simulink library "LibDBC_SCU_ch1"  (R2024b)
settings: Solver=VariableStepAuto  StartTime=0.0  StopTime=10.0  RelTol=1e-3
undefined symbols (not defined in the file): bit_packing, bit_unpacking, IO_Blk_Lib_TTC500, IO_CAN_ConfigMsg, IO_CAN_ReadMsg
libraries: simulink x59, IOBlock_Library_TTC580 x32
(part 16 of 21)

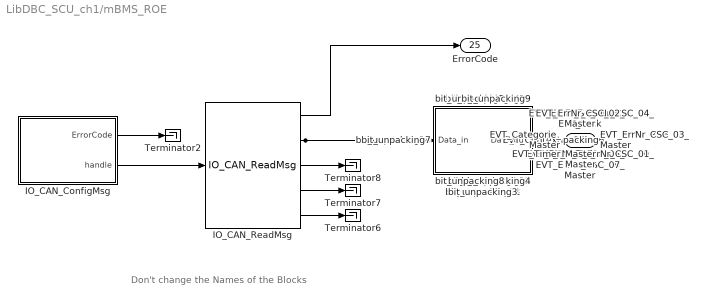
== system LibDBC_SCU_ch1/mBMS_ROE ==
  note: Don't change the Names of the Blocks
  IO_CAN_ConfigMsg : Subsystem  mask(IO_CAN_ConfigMsg_Code){SampleTime=-1, ttlib=IO_Blk_Lib_TTC500, ttDescription=IO_CAN_ConfigMsg, tt_iolib_version=0.19, channel=IO_CAN_CHANNEL_1, mode=IO_CAN_MSG_READ, id_format=IO_CAN_STD_FRAME, id=0x102, ac_mask=0x7FF}
      mask help: Configures a message object for the given CAN channel.
      mask init:
      | %
      mask Help: web(which('IO_CAN.h'))
      mask TypeOptions channel: IO_CAN_CHANNEL_0  | IO_CAN_CHANNEL_1 | IO_CAN_CHANNEL_2 | IO_CAN_CHANNEL_3 | IO_CAN_CHANNEL_4 | IO_CAN_CHANNEL_5 | IO_CAN_CHANNEL_6
      mask Callback channel: %
      mask TypeOptions mode: IO_CAN_MSG_READ | IO_CAN_MSG_WRITE
      mask Callback mode: %
      mask TypeOptions id_format: IO_CAN_STD_FRAME | IO_CAN_EXT_FRAME
      mask Callback id_format: %
      mask Callback id: %
      mask Callback ac_mask: %
  IO_CAN_ReadMsg : IOBlock_Library_TTC580/CAN  Blocks TTC580 IOlib/ReadMsg_CAN/IO_CAN_ReadMsg  SampleTime=-1  ttlib=IO_Blk_Lib_TTC500  ttDescription=IO_CAN_ReadMsg  tt_iolib_version=0.19
      settings: SourceProductName=I/O Blocklibrary for TTC580
  Terminator{2,6..8} (4 alike) : Terminator
  bit_unpacking1 : Subsystem  LoadFcn=|  mask(bit_unpacking_Code){SampleTime=-1, ttlib=IO_Blk_Lib_TTC500, ttDescription=bit_unpacking, tt_iolib_version=0.26, Endianness=little, Format=unsigned, Inversion=off, Startbit=0, Width_bits=5, Factor=1, Offset=0}
      | try
      | %
      | %Upgrade Information - standard BEGIN
      | new_color = 'blue';
      | new_ver = '0.26';
      | act_ver = get_param(gcb,'tt_iolib_version');
      | if not(strcmp(act_ver,new_ver))
      |     disp(['Upgrade block: ',gcb,char(10),'       Version: ',act_ver,' to ',new_ver]);
      |     %switch - case for specific upgrade information e.g. additional parameter required 
      |     %Change appearance and version information
      |     set_param(gcb,'ForegroundColor',new_color);
      |     set_param(gcb,'tt_iolib_version',new_ver);
      | end
      | %Upgrade Information - standard END
      | catch
      | %Standard catch section BEGIN
      | errordlg('An error occurred in a callback of the TTC580-BlockLib. Please open the Diagnostic Viewer for further details');
      | disp(' ');
      | disp('------------------------------------------------------------');
      | disp('An error occurred in a callback of the TTC580-BlockLib.');
      | disp(['Please check the parameters in the mask of ',gcb]);
      | disp('If you do not encounter any violations, then please '); 
      | disp('copy the following lines and report this to support@ttcontrol.com ');
      | disp('<< begin of error message dump >>');
      | disp(['Version of TTC580-BlockLib: ', get_param(gcb,'tt_iolib_version')]);
      | disp(get_param(gcb,'ttDescription'));
      | disp(gcb);
      | x=lasterror;disp(x.message);
      | disp(get_param(gcb,'MaskValues'));
      | disp(version);
      | disp(computer);
      | disp('<< end of error message dump >>');
      | disp('------------------------------------------------------------');
      | disp(' ');
      | %Standard catch section END
      | end
      mask help:
      | Block to read in CAN signal from a specified position within 64bit field.
      | For "Factor" and "Offset" the definition of Vector's CANdb applies:
      | [Physical value] = ( [Raw value] * [Factor] ) + [Offset]
      | with Raw value of a signal being the value as it is transmitted in the CAN-network
      | Verification capabilities are supported.
      mask init: same as LibDBC_SCU_ch1/EXT_BalancingRequest/bit_packing1
      mask Help: web([which('usermanual.html'),'#',lower(get_param(gcb,'ttDescription'))])
      mask TypeOptions Endianness: big | little
      mask Callback Endianness: %
      mask TypeOptions Format: unsigned | signed | real32
      mask Callback Format: %
      mask Callback Inversion: %
      mask Callback Startbit: %
      mask Callback Width_bits: %
      mask Callback Factor: %
      mask Callback Offset: %
  bit_unpacking10 : Subsystem  LoadFcn=|  mask(bit_unpacking_Code){SampleTime=-1, ttlib=IO_Blk_Lib_TTC500, ttDescription=bit_unpacking, tt_iolib_version=0.26, Endianness=little, Format=unsigned, Inversion=off, Startbit=8, Width_bits=8, Factor=1, Offset=0}
      | try
      | %
      | %Upgrade Information - standard BEGIN
      | new_color = 'blue';
      | new_ver = '0.26';
      | act_ver = get_param(gcb,'tt_iolib_version');
      | if not(strcmp(act_ver,new_ver))
      |     disp(['Upgrade block: ',gcb,char(10),'       Version: ',act_ver,' to ',new_ver]);
      |     %switch - case for specific upgrade information e.g. additional parameter required 
      |     %Change appearance and version information
      |     set_param(gcb,'ForegroundColor',new_color);
      |     set_param(gcb,'tt_iolib_version',new_ver);
      | end
      | %Upgrade Information - standard END
      | catch
      | %Standard catch section BEGIN
      | errordlg('An error occurred in a callback of the TTC580-BlockLib. Please open the Diagnostic Viewer for further details');
      | disp(' ');
      | disp('------------------------------------------------------------');
      | disp('An error occurred in a callback of the TTC580-BlockLib.');
      | disp(['Please check the parameters in the mask of ',gcb]);
      | disp('If you do not encounter any violations, then please '); 
      | disp('copy the following lines and report this to support@ttcontrol.com ');
      | disp('<< begin of error message dump >>');
      | disp(['Version of TTC580-BlockLib: ', get_param(gcb,'tt_iolib_version')]);
      | disp(get_param(gcb,'ttDescription'));
      | disp(gcb);
      | x=lasterror;disp(x.message);
      | disp(get_param(gcb,'MaskValues'));
      | disp(version);
      | disp(computer);
      | disp('<< end of error message dump >>');
      | disp('------------------------------------------------------------');
      | disp(' ');
      | %Standard catch section END
      | end
      mask help:
      | Block to read in CAN signal from a specified position within 64bit field.
      | For "Factor" and "Offset" the definition of Vector's CANdb applies:
      | [Physical value] = ( [Raw value] * [Factor] ) + [Offset]
      | with Raw value of a signal being the value as it is transmitted in the CAN-network
      | Verification capabilities are supported.
      mask init: same as LibDBC_SCU_ch1/EXT_BalancingRequest/bit_packing1
      mask Help: web([which('usermanual.html'),'#',lower(get_param(gcb,'ttDescription'))])
      mask TypeOptions Endianness: big | little
      mask Callback Endianness: %
      mask TypeOptions Format: unsigned | signed | real32
      mask Callback Format: %
      mask Callback Inversion: %
      mask Callback Startbit: %
      mask Callback Width_bits: %
      mask Callback Factor: %
      mask Callback Offset: %
  bit_unpacking11 : Subsystem  LoadFcn=|  mask(bit_unpacking_Code){SampleTime=-1, ttlib=IO_Blk_Lib_TTC500, ttDescription=bit_unpacking, tt_iolib_version=0.26, Endianness=little, Format=unsigned, Inversion=off, Startbit=8, Width_bits=8, Factor=1, Offset=0}
      | try
      | %
      | %Upgrade Information - standard BEGIN
      | new_color = 'blue';
      | new_ver = '0.26';
      | act_ver = get_param(gcb,'tt_iolib_version');
      | if not(strcmp(act_ver,new_ver))
      |     disp(['Upgrade block: ',gcb,char(10),'       Version: ',act_ver,' to ',new_ver]);
      |     %switch - case for specific upgrade information e.g. additional parameter required 
      |     %Change appearance and version information
      |     set_param(gcb,'ForegroundColor',new_color);
      |     set_param(gcb,'tt_iolib_version',new_ver);
      | end
      | %Upgrade Information - standard END
      | catch
      | %Standard catch section BEGIN
      | errordlg('An error occurred in a callback of the TTC580-BlockLib. Please open the Diagnostic Viewer for further details');
      | disp(' ');
      | disp('------------------------------------------------------------');
      | disp('An error occurred in a callback of the TTC580-BlockLib.');
      | disp(['Please check the parameters in the mask of ',gcb]);
      | disp('If you do not encounter any violations, then please '); 
      | disp('copy the following lines and report this to support@ttcontrol.com ');
      | disp('<< begin of error message dump >>');
      | disp(['Version of TTC580-BlockLib: ', get_param(gcb,'tt_iolib_version')]);
      | disp(get_param(gcb,'ttDescription'));
      | disp(gcb);
      | x=lasterror;disp(x.message);
      | disp(get_param(gcb,'MaskValues'));
      | disp(version);
      | disp(computer);
      | disp('<< end of error message dump >>');
      | disp('------------------------------------------------------------');
      | disp(' ');
      | %Standard catch section END
      | end
      mask help:
      | Block to read in CAN signal from a specified position within 64bit field.
      | For "Factor" and "Offset" the definition of Vector's CANdb applies:
      | [Physical value] = ( [Raw value] * [Factor] ) + [Offset]
      | with Raw value of a signal being the value as it is transmitted in the CAN-network
      | Verification capabilities are supported.
      mask init: same as LibDBC_SCU_ch1/EXT_BalancingRequest/bit_packing1
      mask Help: web([which('usermanual.html'),'#',lower(get_param(gcb,'ttDescription'))])
      mask TypeOptions Endianness: big | little
      mask Callback Endianness: %
      mask TypeOptions Format: unsigned | signed | real32
      mask Callback Format: %
      mask Callback Inversion: %
      mask Callback Startbit: %
      mask Callback Width_bits: %
      mask Callback Factor: %
      mask Callback Offset: %
  bit_unpacking12 : Subsystem  LoadFcn=|  mask(bit_unpacking_Code){SampleTime=-1, ttlib=IO_Blk_Lib_TTC500, ttDescription=bit_unpacking, tt_iolib_version=0.26, Endianness=little, Format=unsigned, Inversion=off, Startbit=8, Width_bits=8, Factor=1, Offset=0}
      | try
      | %
      | %Upgrade Information - standard BEGIN
      | new_color = 'blue';
      | new_ver = '0.26';
      | act_ver = get_param(gcb,'tt_iolib_version');
      | if not(strcmp(act_ver,new_ver))
      |     disp(['Upgrade block: ',gcb,char(10),'       Version: ',act_ver,' to ',new_ver]);
      |     %switch - case for specific upgrade information e.g. additional parameter required 
      |     %Change appearance and version information
      |     set_param(gcb,'ForegroundColor',new_color);
      |     set_param(gcb,'tt_iolib_version',new_ver);
      | end
      | %Upgrade Information - standard END
      | catch
      | %Standard catch section BEGIN
      | errordlg('An error occurred in a callback of the TTC580-BlockLib. Please open the Diagnostic Viewer for further details');
      | disp(' ');
      | disp('------------------------------------------------------------');
      | disp('An error occurred in a callback of the TTC580-BlockLib.');
      | disp(['Please check the parameters in the mask of ',gcb]);
      | disp('If you do not encounter any violations, then please '); 
      | disp('copy the following lines and report this to support@ttcontrol.com ');
      | disp('<< begin of error message dump >>');
      | disp(['Version of TTC580-BlockLib: ', get_param(gcb,'tt_iolib_version')]);
      | disp(get_param(gcb,'ttDescription'));
      | disp(gcb);
      | x=lasterror;disp(x.message);
      | disp(get_param(gcb,'MaskValues'));
      | disp(version);
      | disp(computer);
      | disp('<< end of error message dump >>');
      | disp('------------------------------------------------------------');
      | disp(' ');
      | %Standard catch section END
      | end
      mask help:
      | Block to read in CAN signal from a specified position within 64bit field.
      | For "Factor" and "Offset" the definition of Vector's CANdb applies:
      | [Physical value] = ( [Raw value] * [Factor] ) + [Offset]
      | with Raw value of a signal being the value as it is transmitted in the CAN-network
      | Verification capabilities are supported.
      mask init: same as LibDBC_SCU_ch1/EXT_BalancingRequest/bit_packing1
      mask Help: web([which('usermanual.html'),'#',lower(get_param(gcb,'ttDescription'))])
      mask TypeOptions Endianness: big | little
      mask Callback Endianness: %
      mask TypeOptions Format: unsigned | signed | real32
      mask Callback Format: %
      mask Callback Inversion: %
      mask Callback Startbit: %
      mask Callback Width_bits: %
      mask Callback Factor: %
      mask Callback Offset: %
  bit_unpacking13 : Subsystem  LoadFcn=|  mask(bit_unpacking_Code){SampleTime=-1, ttlib=IO_Blk_Lib_TTC500, ttDescription=bit_unpacking, tt_iolib_version=0.26, Endianness=little, Format=unsigned, Inversion=off, Startbit=8, Width_bits=8, Factor=1, Offset=0}
      | try
      | %
      | %Upgrade Information - standard BEGIN
      | new_color = 'blue';
      | new_ver = '0.26';
      | act_ver = get_param(gcb,'tt_iolib_version');
      | if not(strcmp(act_ver,new_ver))
      |     disp(['Upgrade block: ',gcb,char(10),'       Version: ',act_ver,' to ',new_ver]);
      |     %switch - case for specific upgrade information e.g. additional parameter required 
      |     %Change appearance and version information
      |     set_param(gcb,'ForegroundColor',new_color);
      |     set_param(gcb,'tt_iolib_version',new_ver);
      | end
      | %Upgrade Information - standard END
      | catch
      | %Standard catch section BEGIN
      | errordlg('An error occurred in a callback of the TTC580-BlockLib. Please open the Diagnostic Viewer for further details');
      | disp(' ');
      | disp('------------------------------------------------------------');
      | disp('An error occurred in a callback of the TTC580-BlockLib.');
      | disp(['Please check the parameters in the mask of ',gcb]);
      | disp('If you do not encounter any violations, then please '); 
      | disp('copy the following lines and report this to support@ttcontrol.com ');
      | disp('<< begin of error message dump >>');
      | disp(['Version of TTC580-BlockLib: ', get_param(gcb,'tt_iolib_version')]);
      | disp(get_param(gcb,'ttDescription'));
      | disp(gcb);
      | x=lasterror;disp(x.message);
      | disp(get_param(gcb,'MaskValues'));
      | disp(version);
      | disp(computer);
      | disp('<< end of error message dump >>');
      | disp('------------------------------------------------------------');
      | disp(' ');
      | %Standard catch section END
      | end
      mask help:
      | Block to read in CAN signal from a specified position within 64bit field.
      | For "Factor" and "Offset" the definition of Vector's CANdb applies:
      | [Physical value] = ( [Raw value] * [Factor] ) + [Offset]
      | with Raw value of a signal being the value as it is transmitted in the CAN-network
      | Verification capabilities are supported.
      mask init: same as LibDBC_SCU_ch1/EXT_BalancingRequest/bit_packing1
      mask Help: web([which('usermanual.html'),'#',lower(get_param(gcb,'ttDescription'))])
      mask TypeOptions Endianness: big | little
      mask Callback Endianness: %
      mask TypeOptions Format: unsigned | signed | real32
      mask Callback Format: %
      mask Callback Inversion: %
      mask Callback Startbit: %
      mask Callback Width_bits: %
      mask Callback Factor: %
      mask Callback Offset: %
  bit_unpacking14 : Subsystem  LoadFcn=|  mask(bit_unpacking_Code){SampleTime=-1, ttlib=IO_Blk_Lib_TTC500, ttDescription=bit_unpacking, tt_iolib_version=0.26, Endianness=little, Format=unsigned, Inversion=off, Startbit=8, Width_bits=8, Factor=1, Offset=0}
      | try
      | %
      | %Upgrade Information - standard BEGIN
      | new_color = 'blue';
      | new_ver = '0.26';
      | act_ver = get_param(gcb,'tt_iolib_version');
      | if not(strcmp(act_ver,new_ver))
      |     disp(['Upgrade block: ',gcb,char(10),'       Version: ',act_ver,' to ',new_ver]);
      |     %switch - case for specific upgrade information e.g. additional parameter required 
      |     %Change appearance and version information
      |     set_param(gcb,'ForegroundColor',new_color);
      |     set_param(gcb,'tt_iolib_version',new_ver);
      | end
      | %Upgrade Information - standard END
      | catch
      | %Standard catch section BEGIN
      | errordlg('An error occurred in a callback of the TTC580-BlockLib. Please open the Diagnostic Viewer for further details');
      | disp(' ');
      | disp('------------------------------------------------------------');
      | disp('An error occurred in a callback of the TTC580-BlockLib.');
      | disp(['Please check the parameters in the mask of ',gcb]);
      | disp('If you do not encounter any violations, then please '); 
      | disp('copy the following lines and report this to support@ttcontrol.com ');
      | disp('<< begin of error message dump >>');
      | disp(['Version of TTC580-BlockLib: ', get_param(gcb,'tt_iolib_version')]);
      | disp(get_param(gcb,'ttDescription'));
      | disp(gcb);
      | x=lasterror;disp(x.message);
      | disp(get_param(gcb,'MaskValues'));
      | disp(version);
      | disp(computer);
      | disp('<< end of error message dump >>');
      | disp('------------------------------------------------------------');
      | disp(' ');
      | %Standard catch section END
      | end
      mask help:
      | Block to read in CAN signal from a specified position within 64bit field.
      | For "Factor" and "Offset" the definition of Vector's CANdb applies:
      | [Physical value] = ( [Raw value] * [Factor] ) + [Offset]
      | with Raw value of a signal being the value as it is transmitted in the CAN-network
      | Verification capabilities are supported.
      mask init: same as LibDBC_SCU_ch1/EXT_BalancingRequest/bit_packing1
      mask Help: web([which('usermanual.html'),'#',lower(get_param(gcb,'ttDescription'))])
      mask TypeOptions Endianness: big | little
      mask Callback Endianness: %
      mask TypeOptions Format: unsigned | signed | real32
      mask Callback Format: %
      mask Callback Inversion: %
      mask Callback Startbit: %
      mask Callback Width_bits: %
      mask Callback Factor: %
      mask Callback Offset: %
  bit_unpacking15 : Subsystem  LoadFcn=|  mask(bit_unpacking_Code){SampleTime=-1, ttlib=IO_Blk_Lib_TTC500, ttDescription=bit_unpacking, tt_iolib_version=0.26, Endianness=little, Format=unsigned, Inversion=off, Startbit=8, Width_bits=8, Factor=1, Offset=0}
      | try
      | %
      | %Upgrade Information - standard BEGIN
      | new_color = 'blue';
      | new_ver = '0.26';
      | act_ver = get_param(gcb,'tt_iolib_version');
      | if not(strcmp(act_ver,new_ver))
      |     disp(['Upgrade block: ',gcb,char(10),'       Version: ',act_ver,' to ',new_ver]);
      |     %switch - case for specific upgrade information e.g. additional parameter required 
      |     %Change appearance and version information
      |     set_param(gcb,'ForegroundColor',new_color);
      |     set_param(gcb,'tt_iolib_version',new_ver);
      | end
      | %Upgrade Information - standard END
      | catch
      | %Standard catch section BEGIN
      | errordlg('An error occurred in a callback of the TTC580-BlockLib. Please open the Diagnostic Viewer for further details');
      | disp(' ');
      | disp('------------------------------------------------------------');
      | disp('An error occurred in a callback of the TTC580-BlockLib.');
      | disp(['Please check the parameters in the mask of ',gcb]);
      | disp('If you do not encounter any violations, then please '); 
      | disp('copy the following lines and report this to support@ttcontrol.com ');
      | disp('<< begin of error message dump >>');
      | disp(['Version of TTC580-BlockLib: ', get_param(gcb,'tt_iolib_version')]);
      | disp(get_param(gcb,'ttDescription'));
      | disp(gcb);
      | x=lasterror;disp(x.message);
      | disp(get_param(gcb,'MaskValues'));
      | disp(version);
      | disp(computer);
      | disp('<< end of error message dump >>');
      | disp('------------------------------------------------------------');
      | disp(' ');
      | %Standard catch section END
      | end
      mask help:
      | Block to read in CAN signal from a specified position within 64bit field.
      | For "Factor" and "Offset" the definition of Vector's CANdb applies:
      | [Physical value] = ( [Raw value] * [Factor] ) + [Offset]
      | with Raw value of a signal being the value as it is transmitted in the CAN-network
      | Verification capabilities are supported.
      mask init: same as LibDBC_SCU_ch1/EXT_BalancingRequest/bit_packing1
      mask Help: web([which('usermanual.html'),'#',lower(get_param(gcb,'ttDescription'))])
      mask TypeOptions Endianness: big | little
      mask Callback Endianness: %
      mask TypeOptions Format: unsigned | signed | real32
      mask Callback Format: %
      mask Callback Inversion: %
      mask Callback Startbit: %
      mask Callback Width_bits: %
      mask Callback Factor: %
      mask Callback Offset: %
  bit_unpacking16 : Subsystem  LoadFcn=|  mask(bit_unpacking_Code){SampleTime=-1, ttlib=IO_Blk_Lib_TTC500, ttDescription=bit_unpacking, tt_iolib_version=0.26, Endianness=little, Format=unsigned, Inversion=off, Startbit=8, Width_bits=8, Factor=1, Offset=0}
      | try
      | %
      | %Upgrade Information - standard BEGIN
      | new_color = 'blue';
      | new_ver = '0.26';
      | act_ver = get_param(gcb,'tt_iolib_version');
      | if not(strcmp(act_ver,new_ver))
      |     disp(['Upgrade block: ',gcb,char(10),'       Version: ',act_ver,' to ',new_ver]);
      |     %switch - case for specific upgrade information e.g. additional parameter required 
      |     %Change appearance and version information
      |     set_param(gcb,'ForegroundColor',new_color);
      |     set_param(gcb,'tt_iolib_version',new_ver);
      | end
      | %Upgrade Information - standard END
      | catch
      | %Standard catch section BEGIN
      | errordlg('An error occurred in a callback of the TTC580-BlockLib. Please open the Diagnostic Viewer for further details');
      | disp(' ');
      | disp('------------------------------------------------------------');
      | disp('An error occurred in a callback of the TTC580-BlockLib.');
      | disp(['Please check the parameters in the mask of ',gcb]);
      | disp('If you do not encounter any violations, then please '); 
      | disp('copy the following lines and report this to support@ttcontrol.com ');
      | disp('<< begin of error message dump >>');
      | disp(['Version of TTC580-BlockLib: ', get_param(gcb,'tt_iolib_version')]);
      | disp(get_param(gcb,'ttDescription'));
      | disp(gcb);
      | x=lasterror;disp(x.message);
      | disp(get_param(gcb,'MaskValues'));
      | disp(version);
      | disp(computer);
      | disp('<< end of error message dump >>');
      | disp('------------------------------------------------------------');
      | disp(' ');
      | %Standard catch section END
      | end
      mask help:
      | Block to read in CAN signal from a specified position within 64bit field.
      | For "Factor" and "Offset" the definition of Vector's CANdb applies:
      | [Physical value] = ( [Raw value] * [Factor] ) + [Offset]
      | with Raw value of a signal being the value as it is transmitted in the CAN-network
      | Verification capabilities are supported.
      mask init: same as LibDBC_SCU_ch1/EXT_BalancingRequest/bit_packing1
      mask Help: web([which('usermanual.html'),'#',lower(get_param(gcb,'ttDescription'))])
      mask TypeOptions Endianness: big | little
      mask Callback Endianness: %
      mask TypeOptions Format: unsigned | signed | real32
      mask Callback Format: %
      mask Callback Inversion: %
      mask Callback Startbit: %
      mask Callback Width_bits: %
      mask Callback Factor: %
      mask Callback Offset: %
  bit_unpacking17 : Subsystem  LoadFcn=|  mask(bit_unpacking_Code){SampleTime=-1, ttlib=IO_Blk_Lib_TTC500, ttDescription=bit_unpacking, tt_iolib_version=0.26, Endianness=little, Format=unsigned, Inversion=off, Startbit=8, Width_bits=8, Factor=1, Offset=0}
      | try
      | %
      | %Upgrade Information - standard BEGIN
      | new_color = 'blue';
      | new_ver = '0.26';
      | act_ver = get_param(gcb,'tt_iolib_version');
      | if not(strcmp(act_ver,new_ver))
      |     disp(['Upgrade block: ',gcb,char(10),'       Version: ',act_ver,' to ',new_ver]);
      |     %switch - case for specific upgrade information e.g. additional parameter required 
      |     %Change appearance and version information
      |     set_param(gcb,'ForegroundColor',new_color);
      |     set_param(gcb,'tt_iolib_version',new_ver);
      | end
      | %Upgrade Information - standard END
      | catch
      | %Standard catch section BEGIN
      | errordlg('An error occurred in a callback of the TTC580-BlockLib. Please open the Diagnostic Viewer for further details');
      | disp(' ');
      | disp('------------------------------------------------------------');
      | disp('An error occurred in a callback of the TTC580-BlockLib.');
      | disp(['Please check the parameters in the mask of ',gcb]);
      | disp('If you do not encounter any violations, then please '); 
      | disp('copy the following lines and report this to support@ttcontrol.com ');
      | disp('<< begin of error message dump >>');
      | disp(['Version of TTC580-BlockLib: ', get_param(gcb,'tt_iolib_version')]);
      | disp(get_param(gcb,'ttDescription'));
      | disp(gcb);
      | x=lasterror;disp(x.message);
      | disp(get_param(gcb,'MaskValues'));
      | disp(version);
      | disp(computer);
      | disp('<< end of error message dump >>');
      | disp('------------------------------------------------------------');
      | disp(' ');
      | %Standard catch section END
      | end
      mask help:
      | Block to read in CAN signal from a specified position within 64bit field.
      | For "Factor" and "Offset" the definition of Vector's CANdb applies:
      | [Physical value] = ( [Raw value] * [Factor] ) + [Offset]
      | with Raw value of a signal being the value as it is transmitted in the CAN-network
      | Verification capabilities are supported.
      mask init: same as LibDBC_SCU_ch1/EXT_BalancingRequest/bit_packing1
      mask Help: web([which('usermanual.html'),'#',lower(get_param(gcb,'ttDescription'))])
      mask TypeOptions Endianness: big | little
      mask Callback Endianness: %
      mask TypeOptions Format: unsigned | signed | real32
      mask Callback Format: %
      mask Callback Inversion: %
      mask Callback Startbit: %
      mask Callback Width_bits: %
      mask Callback Factor: %
      mask Callback Offset: %
  bit_unpacking18 : Subsystem  LoadFcn=|  mask(bit_unpacking_Code){SampleTime=-1, ttlib=IO_Blk_Lib_TTC500, ttDescription=bit_unpacking, tt_iolib_version=0.26, Endianness=little, Format=unsigned, Inversion=off, Startbit=8, Width_bits=8, Factor=1, Offset=0}
      | try
      | %
      | %Upgrade Information - standard BEGIN
      | new_color = 'blue';
      | new_ver = '0.26';
      | act_ver = get_param(gcb,'tt_iolib_version');
      | if not(strcmp(act_ver,new_ver))
      |     disp(['Upgrade block: ',gcb,char(10),'       Version: ',act_ver,' to ',new_ver]);
      |     %switch - case for specific upgrade information e.g. additional parameter required 
      |     %Change appearance and version information
      |     set_param(gcb,'ForegroundColor',new_color);
      |     set_param(gcb,'tt_iolib_version',new_ver);
      | end
      | %Upgrade Information - standard END
      | catch
      | %Standard catch section BEGIN
      | errordlg('An error occurred in a callback of the TTC580-BlockLib. Please open the Diagnostic Viewer for further details');
      | disp(' ');
      | disp('------------------------------------------------------------');
      | disp('An error occurred in a callback of the TTC580-BlockLib.');
      | disp(['Please check the parameters in the mask of ',gcb]);
      | disp('If you do not encounter any violations, then please '); 
      | disp('copy the following lines and report this to support@ttcontrol.com ');
      | disp('<< begin of error message dump >>');
      | disp(['Version of TTC580-BlockLib: ', get_param(gcb,'tt_iolib_version')]);
      | disp(get_param(gcb,'ttDescription'));
      | disp(gcb);
      | x=lasterror;disp(x.message);
      | disp(get_param(gcb,'MaskValues'));
      | disp(version);
      | disp(computer);
      | disp('<< end of error message dump >>');
      | disp('------------------------------------------------------------');
      | disp(' ');
      | %Standard catch section END
      | end
      mask help:
      | Block to read in CAN signal from a specified position within 64bit field.
      | For "Factor" and "Offset" the definition of Vector's CANdb applies:
      | [Physical value] = ( [Raw value] * [Factor] ) + [Offset]
      | with Raw value of a signal being the value as it is transmitted in the CAN-network
      | Verification capabilities are supported.
      mask init: same as LibDBC_SCU_ch1/EXT_BalancingRequest/bit_packing1
      mask Help: web([which('usermanual.html'),'#',lower(get_param(gcb,'ttDescription'))])
      mask TypeOptions Endianness: big | little
      mask Callback Endianness: %
      mask TypeOptions Format: unsigned | signed | real32
      mask Callback Format: %
      mask Callback Inversion: %
      mask Callback Startbit: %
      mask Callback Width_bits: %
      mask Callback Factor: %
      mask Callback Offset: %
  bit_unpacking19 : Subsystem  LoadFcn=|  mask(bit_unpacking_Code){SampleTime=-1, ttlib=IO_Blk_Lib_TTC500, ttDescription=bit_unpacking, tt_iolib_version=0.26, Endianness=little, Format=unsigned, Inversion=off, Startbit=8, Width_bits=8, Factor=1, Offset=0}
      | try
      | %
      | %Upgrade Information - standard BEGIN
      | new_color = 'blue';
      | new_ver = '0.26';
      | act_ver = get_param(gcb,'tt_iolib_version');
      | if not(strcmp(act_ver,new_ver))
      |     disp(['Upgrade block: ',gcb,char(10),'       Version: ',act_ver,' to ',new_ver]);
      |     %switch - case for specific upgrade information e.g. additional parameter required 
      |     %Change appearance and version information
      |     set_param(gcb,'ForegroundColor',new_color);
      |     set_param(gcb,'tt_iolib_version',new_ver);
      | end
      | %Upgrade Information - standard END
      | catch
      | %Standard catch section BEGIN
      | errordlg('An error occurred in a callback of the TTC580-BlockLib. Please open the Diagnostic Viewer for further details');
      | disp(' ');
      | disp('------------------------------------------------------------');
      | disp('An error occurred in a callback of the TTC580-BlockLib.');
      | disp(['Please check the parameters in the mask of ',gcb]);
      | disp('If you do not encounter any violations, then please '); 
      | disp('copy the following lines and report this to support@ttcontrol.com ');
      | disp('<< begin of error message dump >>');
      | disp(['Version of TTC580-BlockLib: ', get_param(gcb,'tt_iolib_version')]);
      | disp(get_param(gcb,'ttDescription'));
      | disp(gcb);
      | x=lasterror;disp(x.message);
      | disp(get_param(gcb,'MaskValues'));
      | disp(version);
      | disp(computer);
      | disp('<< end of error message dump >>');
      | disp('------------------------------------------------------------');
      | disp(' ');
      | %Standard catch section END
      | end
      mask help:
      | Block to read in CAN signal from a specified position within 64bit field.
      | For "Factor" and "Offset" the definition of Vector's CANdb applies:
      | [Physical value] = ( [Raw value] * [Factor] ) + [Offset]
      | with Raw value of a signal being the value as it is transmitted in the CAN-network
      | Verification capabilities are supported.
      mask init: same as LibDBC_SCU_ch1/EXT_BalancingRequest/bit_packing1
      mask Help: web([which('usermanual.html'),'#',lower(get_param(gcb,'ttDescription'))])
      mask TypeOptions Endianness: big | little
      mask Callback Endianness: %
      mask TypeOptions Format: unsigned | signed | real32
      mask Callback Format: %
      mask Callback Inversion: %
      mask Callback Startbit: %
      mask Callback Width_bits: %
      mask Callback Factor: %
      mask Callback Offset: %
  bit_unpacking2 : Subsystem  LoadFcn=|  mask(bit_unpacking_Code){SampleTime=-1, ttlib=IO_Blk_Lib_TTC500, ttDescription=bit_unpacking, tt_iolib_version=0.26, Endianness=little, Format=unsigned, Inversion=off, Startbit=5, Width_bits=3, Factor=1, Offset=0}
      | try
      | %
      | %Upgrade Information - standard BEGIN
      | new_color = 'blue';
      | new_ver = '0.26';
      | act_ver = get_param(gcb,'tt_iolib_version');
      | if not(strcmp(act_ver,new_ver))
      |     disp(['Upgrade block: ',gcb,char(10),'       Version: ',act_ver,' to ',new_ver]);
      |     %switch - case for specific upgrade information e.g. additional parameter required 
      |     %Change appearance and version information
      |     set_param(gcb,'ForegroundColor',new_color);
      |     set_param(gcb,'tt_iolib_version',new_ver);
      | end
      | %Upgrade Information - standard END
      | catch
      | %Standard catch section BEGIN
      | errordlg('An error occurred in a callback of the TTC580-BlockLib. Please open the Diagnostic Viewer for further details');
      | disp(' ');
      | disp('------------------------------------------------------------');
      | disp('An error occurred in a callback of the TTC580-BlockLib.');
      | disp(['Please check the parameters in the mask of ',gcb]);
      | disp('If you do not encounter any violations, then please '); 
      | disp('copy the following lines and report this to support@ttcontrol.com ');
      | disp('<< begin of error message dump >>');
      | disp(['Version of TTC580-BlockLib: ', get_param(gcb,'tt_iolib_version')]);
      | disp(get_param(gcb,'ttDescription'));
      | disp(gcb);
      | x=lasterror;disp(x.message);
      | disp(get_param(gcb,'MaskValues'));
      | disp(version);
      | disp(computer);
      | disp('<< end of error message dump >>');
      | disp('------------------------------------------------------------');
      | disp(' ');
      | %Standard catch section END
      | end
      mask help:
      | Block to read in CAN signal from a specified position within 64bit field.
      | For "Factor" and "Offset" the definition of Vector's CANdb applies:
      | [Physical value] = ( [Raw value] * [Factor] ) + [Offset]
      | with Raw value of a signal being the value as it is transmitted in the CAN-network
      | Verification capabilities are supported.
      mask init: same as LibDBC_SCU_ch1/EXT_BalancingRequest/bit_packing1
      mask Help: web([which('usermanual.html'),'#',lower(get_param(gcb,'ttDescription'))])
      mask TypeOptions Endianness: big | little
      mask Callback Endianness: %
      mask TypeOptions Format: unsigned | signed | real32
      mask Callback Format: %
      mask Callback Inversion: %
      mask Callback Startbit: %
      mask Callback Width_bits: %
      mask Callback Factor: %
      mask Callback Offset: %
  bit_unpacking20 : Subsystem  LoadFcn=|  mask(bit_unpacking_Code){SampleTime=-1, ttlib=IO_Blk_Lib_TTC500, ttDescription=bit_unpacking, tt_iolib_version=0.26, Endianness=little, Format=unsigned, Inversion=off, Startbit=8, Width_bits=8, Factor=1, Offset=0}
      | try
      | %
      | %Upgrade Information - standard BEGIN
      | new_color = 'blue';
      | new_ver = '0.26';
      | act_ver = get_param(gcb,'tt_iolib_version');
      | if not(strcmp(act_ver,new_ver))
      |     disp(['Upgrade block: ',gcb,char(10),'       Version: ',act_ver,' to ',new_ver]);
      |     %switch - case for specific upgrade information e.g. additional parameter required 
      |     %Change appearance and version information
      |     set_param(gcb,'ForegroundColor',new_color);
      |     set_param(gcb,'tt_iolib_version',new_ver);
      | end
      | %Upgrade Information - standard END
      | catch
      | %Standard catch section BEGIN
      | errordlg('An error occurred in a callback of the TTC580-BlockLib. Please open the Diagnostic Viewer for further details');
      | disp(' ');
      | disp('------------------------------------------------------------');
      | disp('An error occurred in a callback of the TTC580-BlockLib.');
      | disp(['Please check the parameters in the mask of ',gcb]);
      | disp('If you do not encounter any violations, then please '); 
      | disp('copy the following lines and report this to support@ttcontrol.com ');
      | disp('<< begin of error message dump >>');
      | disp(['Version of TTC580-BlockLib: ', get_param(gcb,'tt_iolib_version')]);
      | disp(get_param(gcb,'ttDescription'));
      | disp(gcb);
      | x=lasterror;disp(x.message);
      | disp(get_param(gcb,'MaskValues'));
      | disp(version);
      | disp(computer);
      | disp('<< end of error message dump >>');
      | disp('------------------------------------------------------------');
      | disp(' ');
      | %Standard catch section END
      | end
      mask help:
      | Block to read in CAN signal from a specified position within 64bit field.
      | For "Factor" and "Offset" the definition of Vector's CANdb applies:
      | [Physical value] = ( [Raw value] * [Factor] ) + [Offset]
      | with Raw value of a signal being the value as it is transmitted in the CAN-network
      | Verification capabilities are supported.
      mask init: same as LibDBC_SCU_ch1/EXT_BalancingRequest/bit_packing1
      mask Help: web([which('usermanual.html'),'#',lower(get_param(gcb,'ttDescription'))])
      mask TypeOptions Endianness: big | little
      mask Callback Endianness: %
      mask TypeOptions Format: unsigned | signed | real32
      mask Callback Format: %
      mask Callback Inversion: %
      mask Callback Startbit: %
      mask Callback Width_bits: %
      mask Callback Factor: %
      mask Callback Offset: %
  bit_unpacking21 : Subsystem  LoadFcn=|  mask(bit_unpacking_Code){SampleTime=-1, ttlib=IO_Blk_Lib_TTC500, ttDescription=bit_unpacking, tt_iolib_version=0.26, Endianness=little, Format=unsigned, Inversion=off, Startbit=8, Width_bits=8, Factor=1, Offset=0}
      | try
      | %
      | %Upgrade Information - standard BEGIN
      | new_color = 'blue';
      | new_ver = '0.26';
      | act_ver = get_param(gcb,'tt_iolib_version');
      | if not(strcmp(act_ver,new_ver))
      |     disp(['Upgrade block: ',gcb,char(10),'       Version: ',act_ver,' to ',new_ver]);
      |     %switch - case for specific upgrade information e.g. additional parameter required 
      |     %Change appearance and version information
      |     set_param(gcb,'ForegroundColor',new_color);
      |     set_param(gcb,'tt_iolib_version',new_ver);
      | end
      | %Upgrade Information - standard END
      | catch
      | %Standard catch section BEGIN
      | errordlg('An error occurred in a callback of the TTC580-BlockLib. Please open the Diagnostic Viewer for further details');
      | disp(' ');
      | disp('------------------------------------------------------------');
      | disp('An error occurred in a callback of the TTC580-BlockLib.');
      | disp(['Please check the parameters in the mask of ',gcb]);
      | disp('If you do not encounter any violations, then please '); 
      | disp('copy the following lines and report this to support@ttcontrol.com ');
      | disp('<< begin of error message dump >>');
      | disp(['Version of TTC580-BlockLib: ', get_param(gcb,'tt_iolib_version')]);
      | disp(get_param(gcb,'ttDescription'));
      | disp(gcb);
      | x=lasterror;disp(x.message);
      | disp(get_param(gcb,'MaskValues'));
      | disp(version);
      | disp(computer);
      | disp('<< end of error message dump >>');
      | disp('------------------------------------------------------------');
      | disp(' ');
      | %Standard catch section END
      | end
      mask help:
      | Block to read in CAN signal from a specified position within 64bit field.
      | For "Factor" and "Offset" the definition of Vector's CANdb applies:
      | [Physical value] = ( [Raw value] * [Factor] ) + [Offset]
      | with Raw value of a signal being the value as it is transmitted in the CAN-network
      | Verification capabilities are supported.
      mask init: same as LibDBC_SCU_ch1/EXT_BalancingRequest/bit_packing1
      mask Help: web([which('usermanual.html'),'#',lower(get_param(gcb,'ttDescription'))])
      mask TypeOptions Endianness: big | little
      mask Callback Endianness: %
      mask TypeOptions Format: unsigned | signed | real32
      mask Callback Format: %
      mask Callback Inversion: %
      mask Callback Startbit: %
      mask Callback Width_bits: %
      mask Callback Factor: %
      mask Callback Offset: %
  bit_unpacking22 : Subsystem  LoadFcn=|  mask(bit_unpacking_Code){SampleTime=-1, ttlib=IO_Blk_Lib_TTC500, ttDescription=bit_unpacking, tt_iolib_version=0.26, Endianness=little, Format=signed, Inversion=off, Startbit=16, Width_bits=16, Factor=1, Offset=0}
      | try
      | %
      | %Upgrade Information - standard BEGIN
      | new_color = 'blue';
      | new_ver = '0.26';
      | act_ver = get_param(gcb,'tt_iolib_version');
      | if not(strcmp(act_ver,new_ver))
      |     disp(['Upgrade block: ',gcb,char(10),'       Version: ',act_ver,' to ',new_ver]);
      |     %switch - case for specific upgrade information e.g. additional parameter required 
      |     %Change appearance and version information
      |     set_param(gcb,'ForegroundColor',new_color);
      |     set_param(gcb,'tt_iolib_version',new_ver);
      | end
      | %Upgrade Information - standard END
      | catch
      | %Standard catch section BEGIN
      | errordlg('An error occurred in a callback of the TTC580-BlockLib. Please open the Diagnostic Viewer for further details');
      | disp(' ');
      | disp('------------------------------------------------------------');
      | disp('An error occurred in a callback of the TTC580-BlockLib.');
      | disp(['Please check the parameters in the mask of ',gcb]);
      | disp('If you do not encounter any violations, then please '); 
      | disp('copy the following lines and report this to support@ttcontrol.com ');
      | disp('<< begin of error message dump >>');
      | disp(['Version of TTC580-BlockLib: ', get_param(gcb,'tt_iolib_version')]);
      | disp(get_param(gcb,'ttDescription'));
      | disp(gcb);
      | x=lasterror;disp(x.message);
      | disp(get_param(gcb,'MaskValues'));
      | disp(version);
      | disp(computer);
      | disp('<< end of error message dump >>');
      | disp('------------------------------------------------------------');
      | disp(' ');
      | %Standard catch section END
      | end
      mask help:
      | Block to read in CAN signal from a specified position within 64bit field.
      | For "Factor" and "Offset" the definition of Vector's CANdb applies:
      | [Physical value] = ( [Raw value] * [Factor] ) + [Offset]
      | with Raw value of a signal being the value as it is transmitted in the CAN-network
      | Verification capabilities are supported.
      mask init: same as LibDBC_SCU_ch1/EXT_BalancingRequest/bit_packing1
      mask Help: web([which('usermanual.html'),'#',lower(get_param(gcb,'ttDescription'))])
      mask TypeOptions Endianness: big | little
      mask Callback Endianness: %
      mask TypeOptions Format: unsigned | signed | real32
      mask Callback Format: %
      mask Callback Inversion: %
      mask Callback Startbit: %
      mask Callback Width_bits: %
      mask Callback Factor: %
      mask Callback Offset: %
  bit_unpacking23 : Subsystem  LoadFcn=|  mask(bit_unpacking_Code){SampleTime=-1, ttlib=IO_Blk_Lib_TTC500, ttDescription=bit_unpacking, tt_iolib_version=0.26, Endianness=little, Format=unsigned, Inversion=off, Startbit=32, Width_bits=2, Factor=1, Offset=0}
      | try
      | %
      | %Upgrade Information - standard BEGIN
      | new_color = 'blue';
      | new_ver = '0.26';
      | act_ver = get_param(gcb,'tt_iolib_version');
      | if not(strcmp(act_ver,new_ver))
      |     disp(['Upgrade block: ',gcb,char(10),'       Version: ',act_ver,' to ',new_ver]);
      |     %switch - case for specific upgrade information e.g. additional parameter required 
      |     %Change appearance and version information
      |     set_param(gcb,'ForegroundColor',new_color);
      |     set_param(gcb,'tt_iolib_version',new_ver);
      | end
      | %Upgrade Information - standard END
      | catch
      | %Standard catch section BEGIN
      | errordlg('An error occurred in a callback of the TTC580-BlockLib. Please open the Diagnostic Viewer for further details');
      | disp(' ');
      | disp('------------------------------------------------------------');
      | disp('An error occurred in a callback of the TTC580-BlockLib.');
      | disp(['Please check the parameters in the mask of ',gcb]);
      | disp('If you do not encounter any violations, then please '); 
      | disp('copy the following lines and report this to support@ttcontrol.com ');
      | disp('<< begin of error message dump >>');
      | disp(['Version of TTC580-BlockLib: ', get_param(gcb,'tt_iolib_version')]);
      | disp(get_param(gcb,'ttDescription'));
      | disp(gcb);
      | x=lasterror;disp(x.message);
      | disp(get_param(gcb,'MaskValues'));
      | disp(version);
      | disp(computer);
      | disp('<< end of error message dump >>');
      | disp('------------------------------------------------------------');
      | disp(' ');
      | %Standard catch section END
      | end
      mask help:
      | Block to read in CAN signal from a specified position within 64bit field.
      | For "Factor" and "Offset" the definition of Vector's CANdb applies:
      | [Physical value] = ( [Raw value] * [Factor] ) + [Offset]
      | with Raw value of a signal being the value as it is transmitted in the CAN-network
      | Verification capabilities are supported.
      mask init: same as LibDBC_SCU_ch1/EXT_BalancingRequest/bit_packing1
      mask Help: web([which('usermanual.html'),'#',lower(get_param(gcb,'ttDescription'))])
      mask TypeOptions Endianness: big | little
      mask Callback Endianness: %
      mask TypeOptions Format: unsigned | signed | real32
      mask Callback Format: %
      mask Callback Inversion: %
      mask Callback Startbit: %
      mask Callback Width_bits: %
      mask Callback Factor: %
      mask Callback Offset: %
  bit_unpacking24 : Subsystem  LoadFcn=|  mask(bit_unpacking_Code){SampleTime=-1, ttlib=IO_Blk_Lib_TTC500, ttDescription=bit_unpacking, tt_iolib_version=0.26, Endianness=little, Format=unsigned, Inversion=off, Startbit=34, Width_bits=30, Factor=1, Offset=0}
      | try
      | %
      | %Upgrade Information - standard BEGIN
      | new_color = 'blue';
      | new_ver = '0.26';
      | act_ver = get_param(gcb,'tt_iolib_version');
      | if not(strcmp(act_ver,new_ver))
      |     disp(['Upgrade block: ',gcb,char(10),'       Version: ',act_ver,' to ',new_ver]);
      |     %switch - case for specific upgrade information e.g. additional parameter required 
      |     %Change appearance and version information
      |     set_param(gcb,'ForegroundColor',new_color);
      |     set_param(gcb,'tt_iolib_version',new_ver);
      | end
      | %Upgrade Information - standard END
      | catch
      | %Standard catch section BEGIN
      | errordlg('An error occurred in a callback of the TTC580-BlockLib. Please open the Diagnostic Viewer for further details');
      | disp(' ');
      | disp('------------------------------------------------------------');
      | disp('An error occurred in a callback of the TTC580-BlockLib.');
      | disp(['Please check the parameters in the mask of ',gcb]);
      | disp('If you do not encounter any violations, then please '); 
      | disp('copy the following lines and report this to support@ttcontrol.com ');
      | disp('<< begin of error message dump >>');
      | disp(['Version of TTC580-BlockLib: ', get_param(gcb,'tt_iolib_version')]);
      | disp(get_param(gcb,'ttDescription'));
      | disp(gcb);
      | x=lasterror;disp(x.message);
      | disp(get_param(gcb,'MaskValues'));
      | disp(version);
      | disp(computer);
      | disp('<< end of error message dump >>');
      | disp('------------------------------------------------------------');
      | disp(' ');
      | %Standard catch section END
      | end
      mask help:
      | Block to read in CAN signal from a specified position within 64bit field.
      | For "Factor" and "Offset" the definition of Vector's CANdb applies:
      | [Physical value] = ( [Raw value] * [Factor] ) + [Offset]
      | with Raw value of a signal being the value as it is transmitted in the CAN-network
      | Verification capabilities are supported.
      mask init: same as LibDBC_SCU_ch1/EXT_BalancingRequest/bit_packing1
      mask Help: web([which('usermanual.html'),'#',lower(get_param(gcb,'ttDescription'))])
      mask TypeOptions Endianness: big | little
      mask Callback Endianness: %
      mask TypeOptions Format: unsigned | signed | real32
      mask Callback Format: %
      mask Callback Inversion: %
      mask Callback Startbit: %
      mask Callback Width_bits: %
      mask Callback Factor: %
      mask Callback Offset: %
  bit_unpacking3 : Subsystem  LoadFcn=|  mask(bit_unpacking_Code){SampleTime=-1, ttlib=IO_Blk_Lib_TTC500, ttDescription=bit_unpacking, tt_iolib_version=0.26, Endianness=little, Format=unsigned, Inversion=off, Startbit=8, Width_bits=8, Factor=1, Offset=0}
      | try
      | %
      | %Upgrade Information - standard BEGIN
      | new_color = 'blue';
      | new_ver = '0.26';
      | act_ver = get_param(gcb,'tt_iolib_version');
      | if not(strcmp(act_ver,new_ver))
      |     disp(['Upgrade block: ',gcb,char(10),'       Version: ',act_ver,' to ',new_ver]);
      |     %switch - case for specific upgrade information e.g. additional parameter required 
      |     %Change appearance and version information
      |     set_param(gcb,'ForegroundColor',new_color);
      |     set_param(gcb,'tt_iolib_version',new_ver);
      | end
      | %Upgrade Information - standard END
      | catch
      | %Standard catch section BEGIN
      | errordlg('An error occurred in a callback of the TTC580-BlockLib. Please open the Diagnostic Viewer for further details');
      | disp(' ');
      | disp('------------------------------------------------------------');
      | disp('An error occurred in a callback of the TTC580-BlockLib.');
      | disp(['Please check the parameters in the mask of ',gcb]);
      | disp('If you do not encounter any violations, then please '); 
      | disp('copy the following lines and report this to support@ttcontrol.com ');
      | disp('<< begin of error message dump >>');
      | disp(['Version of TTC580-BlockLib: ', get_param(gcb,'tt_iolib_version')]);
      | disp(get_param(gcb,'ttDescription'));
      | disp(gcb);
      | x=lasterror;disp(x.message);
      | disp(get_param(gcb,'MaskValues'));
      | disp(version);
      | disp(computer);
      | disp('<< end of error message dump >>');
      | disp('------------------------------------------------------------');
      | disp(' ');
      | %Standard catch section END
      | end
      mask help:
      | Block to read in CAN signal from a specified position within 64bit field.
      | For "Factor" and "Offset" the definition of Vector's CANdb applies:
      | [Physical value] = ( [Raw value] * [Factor] ) + [Offset]
      | with Raw value of a signal being the value as it is transmitted in the CAN-network
      | Verification capabilities are supported.
      mask init: same as LibDBC_SCU_ch1/EXT_BalancingRequest/bit_packing1
      mask Help: web([which('usermanual.html'),'#',lower(get_param(gcb,'ttDescription'))])
      mask TypeOptions Endianness: big | little
      mask Callback Endianness: %
      mask TypeOptions Format: unsigned | signed | real32
      mask Callback Format: %
      mask Callback Inversion: %
      mask Callback Startbit: %
      mask Callback Width_bits: %
      mask Callback Factor: %
      mask Callback Offset: %
  bit_unpacking4 : Subsystem  LoadFcn=|  mask(bit_unpacking_Code){SampleTime=-1, ttlib=IO_Blk_Lib_TTC500, ttDescription=bit_unpacking, tt_iolib_version=0.26, Endianness=little, Format=unsigned, Inversion=off, Startbit=8, Width_bits=8, Factor=1, Offset=0}
      | try
      | %
      | %Upgrade Information - standard BEGIN
      | new_color = 'blue';
      | new_ver = '0.26';
      | act_ver = get_param(gcb,'tt_iolib_version');
      | if not(strcmp(act_ver,new_ver))
      |     disp(['Upgrade block: ',gcb,char(10),'       Version: ',act_ver,' to ',new_ver]);
      |     %switch - case for specific upgrade information e.g. additional parameter required 
      |     %Change appearance and version information
      |     set_param(gcb,'ForegroundColor',new_color);
      |     set_param(gcb,'tt_iolib_version',new_ver);
      | end
      | %Upgrade Information - standard END
      | catch
      | %Standard catch section BEGIN
      | errordlg('An error occurred in a callback of the TTC580-BlockLib. Please open the Diagnostic Viewer for further details');
      | disp(' ');
      | disp('------------------------------------------------------------');
      | disp('An error occurred in a callback of the TTC580-BlockLib.');
      | disp(['Please check the parameters in the mask of ',gcb]);
      | disp('If you do not encounter any violations, then please '); 
      | disp('copy the following lines and report this to support@ttcontrol.com ');
      | disp('<< begin of error message dump >>');
      | disp(['Version of TTC580-BlockLib: ', get_param(gcb,'tt_iolib_version')]);
      | disp(get_param(gcb,'ttDescription'));
      | disp(gcb);
      | x=lasterror;disp(x.message);
      | disp(get_param(gcb,'MaskValues'));
      | disp(version);
      | disp(computer);
      | disp('<< end of error message dump >>');
      | disp('------------------------------------------------------------');
      | disp(' ');
      | %Standard catch section END
      | end
      mask help:
      | Block to read in CAN signal from a specified position within 64bit field.
      | For "Factor" and "Offset" the definition of Vector's CANdb applies:
      | [Physical value] = ( [Raw value] * [Factor] ) + [Offset]
      | with Raw value of a signal being the value as it is transmitted in the CAN-network
      | Verification capabilities are supported.
      mask init: same as LibDBC_SCU_ch1/EXT_BalancingRequest/bit_packing1
      mask Help: web([which('usermanual.html'),'#',lower(get_param(gcb,'ttDescription'))])
      mask TypeOptions Endianness: big | little
      mask Callback Endianness: %
      mask TypeOptions Format: unsigned | signed | real32
      mask Callback Format: %
      mask Callback Inversion: %
      mask Callback Startbit: %
      mask Callback Width_bits: %
      mask Callback Factor: %
      mask Callback Offset: %
  bit_unpacking5 : Subsystem  LoadFcn=|  mask(bit_unpacking_Code){SampleTime=-1, ttlib=IO_Blk_Lib_TTC500, ttDescription=bit_unpacking, tt_iolib_version=0.26, Endianness=little, Format=unsigned, Inversion=off, Startbit=8, Width_bits=8, Factor=1, Offset=0}
      | try
      | %
      | %Upgrade Information - standard BEGIN
      | new_color = 'blue';
      | new_ver = '0.26';
      | act_ver = get_param(gcb,'tt_iolib_version');
      | if not(strcmp(act_ver,new_ver))
      |     disp(['Upgrade block: ',gcb,char(10),'       Version: ',act_ver,' to ',new_ver]);
      |     %switch - case for specific upgrade information e.g. additional parameter required 
      |     %Change appearance and version information
      |     set_param(gcb,'ForegroundColor',new_color);
      |     set_param(gcb,'tt_iolib_version',new_ver);
      | end
      | %Upgrade Information - standard END
      | catch
      | %Standard catch section BEGIN
      | errordlg('An error occurred in a callback of the TTC580-BlockLib. Please open the Diagnostic Viewer for further details');
      | disp(' ');
      | disp('------------------------------------------------------------');
      | disp('An error occurred in a callback of the TTC580-BlockLib.');
      | disp(['Please check the parameters in the mask of ',gcb]);
      | disp('If you do not encounter any violations, then please '); 
      | disp('copy the following lines and report this to support@ttcontrol.com ');
      | disp('<< begin of error message dump >>');
      | disp(['Version of TTC580-BlockLib: ', get_param(gcb,'tt_iolib_version')]);
      | disp(get_param(gcb,'ttDescription'));
      | disp(gcb);
      | x=lasterror;disp(x.message);
      | disp(get_param(gcb,'MaskValues'));
      | disp(version);
      | disp(computer);
      | disp('<< end of error message dump >>');
      | disp('------------------------------------------------------------');
      | disp(' ');
      | %Standard catch section END
      | end
      mask help:
      | Block to read in CAN signal from a specified position within 64bit field.
      | For "Factor" and "Offset" the definition of Vector's CANdb applies:
      | [Physical value] = ( [Raw value] * [Factor] ) + [Offset]
      | with Raw value of a signal being the value as it is transmitted in the CAN-network
      | Verification capabilities are supported.
      mask init: same as LibDBC_SCU_ch1/EXT_BalancingRequest/bit_packing1
      mask Help: web([which('usermanual.html'),'#',lower(get_param(gcb,'ttDescription'))])
      mask TypeOptions Endianness: big | little
      mask Callback Endianness: %
      mask TypeOptions Format: unsigned | signed | real32
      mask Callback Format: %
      mask Callback Inversion: %
      mask Callback Startbit: %
      mask Callback Width_bits: %
      mask Callback Factor: %
      mask Callback Offset: %
  bit_unpacking6 : Subsystem  LoadFcn=|  mask(bit_unpacking_Code){SampleTime=-1, ttlib=IO_Blk_Lib_TTC500, ttDescription=bit_unpacking, tt_iolib_version=0.26, Endianness=little, Format=unsigned, Inversion=off, Startbit=8, Width_bits=8, Factor=1, Offset=0}
      | try
      | %
      | %Upgrade Information - standard BEGIN
      | new_color = 'blue';
      | new_ver = '0.26';
      | act_ver = get_param(gcb,'tt_iolib_version');
      | if not(strcmp(act_ver,new_ver))
      |     disp(['Upgrade block: ',gcb,char(10),'       Version: ',act_ver,' to ',new_ver]);
      |     %switch - case for specific upgrade information e.g. additional parameter required 
      |     %Change appearance and version information
      |     set_param(gcb,'ForegroundColor',new_color);
      |     set_param(gcb,'tt_iolib_version',new_ver);
      | end
      | %Upgrade Information - standard END
      | catch
      | %Standard catch section BEGIN
      | errordlg('An error occurred in a callback of the TTC580-BlockLib. Please open the Diagnostic Viewer for further details');
      | disp(' ');
      | disp('------------------------------------------------------------');
      | disp('An error occurred in a callback of the TTC580-BlockLib.');
      | disp(['Please check the parameters in the mask of ',gcb]);
      | disp('If you do not encounter any violations, then please '); 
      | disp('copy the following lines and report this to support@ttcontrol.com ');
      | disp('<< begin of error message dump >>');
      | disp(['Version of TTC580-BlockLib: ', get_param(gcb,'tt_iolib_version')]);
      | disp(get_param(gcb,'ttDescription'));
      | disp(gcb);
      | x=lasterror;disp(x.message);
      | disp(get_param(gcb,'MaskValues'));
      | disp(version);
      | disp(computer);
      | disp('<< end of error message dump >>');
      | disp('------------------------------------------------------------');
      | disp(' ');
      | %Standard catch section END
      | end
      mask help:
      | Block to read in CAN signal from a specified position within 64bit field.
      | For "Factor" and "Offset" the definition of Vector's CANdb applies:
      | [Physical value] = ( [Raw value] * [Factor] ) + [Offset]
      | with Raw value of a signal being the value as it is transmitted in the CAN-network
      | Verification capabilities are supported.
      mask init: same as LibDBC_SCU_ch1/EXT_BalancingRequest/bit_packing1
      mask Help: web([which('usermanual.html'),'#',lower(get_param(gcb,'ttDescription'))])
      mask TypeOptions Endianness: big | little
      mask Callback Endianness: %
      mask TypeOptions Format: unsigned | signed | real32
      mask Callback Format: %
      mask Callback Inversion: %
      mask Callback Startbit: %
      mask Callback Width_bits: %
      mask Callback Factor: %
      mask Callback Offset: %
  bit_unpacking7 : Subsystem  LoadFcn=|  mask(bit_unpacking_Code){SampleTime=-1, ttlib=IO_Blk_Lib_TTC500, ttDescription=bit_unpacking, tt_iolib_version=0.26, Endianness=little, Format=unsigned, Inversion=off, Startbit=8, Width_bits=8, Factor=1, Offset=0}
      | try
      | %
      | %Upgrade Information - standard BEGIN
      | new_color = 'blue';
      | new_ver = '0.26';
      | act_ver = get_param(gcb,'tt_iolib_version');
      | if not(strcmp(act_ver,new_ver))
      |     disp(['Upgrade block: ',gcb,char(10),'       Version: ',act_ver,' to ',new_ver]);
      |     %switch - case for specific upgrade information e.g. additional parameter required 
      |     %Change appearance and version information
      |     set_param(gcb,'ForegroundColor',new_color);
      |     set_param(gcb,'tt_iolib_version',new_ver);
      | end
      | %Upgrade Information - standard END
      | catch
      | %Standard catch section BEGIN
      | errordlg('An error occurred in a callback of the TTC580-BlockLib. Please open the Diagnostic Viewer for further details');
      | disp(' ');
      | disp('------------------------------------------------------------');
      | disp('An error occurred in a callback of the TTC580-BlockLib.');
      | disp(['Please check the parameters in the mask of ',gcb]);
      | disp('If you do not encounter any violations, then please '); 
      | disp('copy the following lines and report this to support@ttcontrol.com ');
      | disp('<< begin of error message dump >>');
      | disp(['Version of TTC580-BlockLib: ', get_param(gcb,'tt_iolib_version')]);
      | disp(get_param(gcb,'ttDescription'));
      | disp(gcb);
      | x=lasterror;disp(x.message);
      | disp(get_param(gcb,'MaskValues'));
      | disp(version);
      | disp(computer);
      | disp('<< end of error message dump >>');
      | disp('------------------------------------------------------------');
      | disp(' ');
      | %Standard catch section END
      | end
      mask help:
      | Block to read in CAN signal from a specified position within 64bit field.
      | For "Factor" and "Offset" the definition of Vector's CANdb applies:
      | [Physical value] = ( [Raw value] * [Factor] ) + [Offset]
      | with Raw value of a signal being the value as it is transmitted in the CAN-network
      | Verification capabilities are supported.
      mask init: same as LibDBC_SCU_ch1/EXT_BalancingRequest/bit_packing1
      mask Help: web([which('usermanual.html'),'#',lower(get_param(gcb,'ttDescription'))])
      mask TypeOptions Endianness: big | little
      mask Callback Endianness: %
      mask TypeOptions Format: unsigned | signed | real32
      mask Callback Format: %
      mask Callback Inversion: %
      mask Callback Startbit: %
      mask Callback Width_bits: %
      mask Callback Factor: %
      mask Callback Offset: %
  bit_unpacking8 : Subsystem  LoadFcn=|  mask(bit_unpacking_Code){SampleTime=-1, ttlib=IO_Blk_Lib_TTC500, ttDescription=bit_unpacking, tt_iolib_version=0.26, Endianness=little, Format=unsigned, Inversion=off, Startbit=8, Width_bits=8, Factor=1, Offset=0}
      | try
      | %
      | %Upgrade Information - standard BEGIN
      | new_color = 'blue';
      | new_ver = '0.26';
      | act_ver = get_param(gcb,'tt_iolib_version');
      | if not(strcmp(act_ver,new_ver))
      |     disp(['Upgrade block: ',gcb,char(10),'       Version: ',act_ver,' to ',new_ver]);
      |     %switch - case for specific upgrade information e.g. additional parameter required 
      |     %Change appearance and version information
      |     set_param(gcb,'ForegroundColor',new_color);
      |     set_param(gcb,'tt_iolib_version',new_ver);
      | end
      | %Upgrade Information - standard END
      | catch
      | %Standard catch section BEGIN
      | errordlg('An error occurred in a callback of the TTC580-BlockLib. Please open the Diagnostic Viewer for further details');
      | disp(' ');
      | disp('------------------------------------------------------------');
      | disp('An error occurred in a callback of the TTC580-BlockLib.');
      | disp(['Please check the parameters in the mask of ',gcb]);
      | disp('If you do not encounter any violations, then please '); 
      | disp('copy the following lines and report this to support@ttcontrol.com ');
      | disp('<< begin of error message dump >>');
      | disp(['Version of TTC580-BlockLib: ', get_param(gcb,'tt_iolib_version')]);
      | disp(get_param(gcb,'ttDescription'));
      | disp(gcb);
      | x=lasterror;disp(x.message);
      | disp(get_param(gcb,'MaskValues'));
      | disp(version);
      | disp(computer);
      | disp('<< end of error message dump >>');
      | disp('------------------------------------------------------------');
      | disp(' ');
      | %Standard catch section END
      | end
      mask help:
      | Block to read in CAN signal from a specified position within 64bit field.
      | For "Factor" and "Offset" the definition of Vector's CANdb applies:
      | [Physical value] = ( [Raw value] * [Factor] ) + [Offset]
      | with Raw value of a signal being the value as it is transmitted in the CAN-network
      | Verification capabilities are supported.
      mask init: same as LibDBC_SCU_ch1/EXT_BalancingRequest/bit_packing1
      mask Help: web([which('usermanual.html'),'#',lower(get_param(gcb,'ttDescription'))])
      mask TypeOptions Endianness: big | little
      mask Callback Endianness: %
      mask TypeOptions Format: unsigned | signed | real32
      mask Callback Format: %
      mask Callback Inversion: %
      mask Callback Startbit: %
      mask Callback Width_bits: %
      mask Callback Factor: %
      mask Callback Offset: %
  bit_unpacking9 : Subsystem  LoadFcn=|  mask(bit_unpacking_Code){SampleTime=-1, ttlib=IO_Blk_Lib_TTC500, ttDescription=bit_unpacking, tt_iolib_version=0.26, Endianness=little, Format=unsigned, Inversion=off, Startbit=8, Width_bits=8, Factor=1, Offset=0}
      | try
      | %
      | %Upgrade Information - standard BEGIN
      | new_color = 'blue';
      | new_ver = '0.26';
      | act_ver = get_param(gcb,'tt_iolib_version');
      | if not(strcmp(act_ver,new_ver))
      |     disp(['Upgrade block: ',gcb,char(10),'       Version: ',act_ver,' to ',new_ver]);
      |     %switch - case for specific upgrade information e.g. additional parameter required 
      |     %Change appearance and version information
      |     set_param(gcb,'ForegroundColor',new_color);
      |     set_param(gcb,'tt_iolib_version',new_ver);
      | end
      | %Upgrade Information - standard END
      | catch
      | %Standard catch section BEGIN
      | errordlg('An error occurred in a callback of the TTC580-BlockLib. Please open the Diagnostic Viewer for further details');
      | disp(' ');
      | disp('------------------------------------------------------------');
      | disp('An error occurred in a callback of the TTC580-BlockLib.');
      | disp(['Please check the parameters in the mask of ',gcb]);
      | disp('If you do not encounter any violations, then please '); 
      | disp('copy the following lines and report this to support@ttcontrol.com ');
      | disp('<< begin of error message dump >>');
      | disp(['Version of TTC580-BlockLib: ', get_param(gcb,'tt_iolib_version')]);
      | disp(get_param(gcb,'ttDescription'));
      | disp(gcb);
      | x=lasterror;disp(x.message);
      | disp(get_param(gcb,'MaskValues'));
      | disp(version);
      | disp(computer);
      | disp('<< end of error message dump >>');
      | disp('------------------------------------------------------------');
      | disp(' ');
      | %Standard catch section END
      | end
      mask help:
      | Block to read in CAN signal from a specified position within 64bit field.
      | For "Factor" and "Offset" the definition of Vector's CANdb applies:
      | [Physical value] = ( [Raw value] * [Factor] ) + [Offset]
      | with Raw value of a signal being the value as it is transmitted in the CAN-network
      | Verification capabilities are supported.
      mask init: same as LibDBC_SCU_ch1/EXT_BalancingRequest/bit_packing1
      mask Help: web([which('usermanual.html'),'#',lower(get_param(gcb,'ttDescription'))])
      mask TypeOptions Endianness: big | little
      mask Callback Endianness: %
      mask TypeOptions Format: unsigned | signed | real32
      mask Callback Format: %
      mask Callback Inversion: %
      mask Callback Startbit: %
      mask Callback Width_bits: %
      mask Callback Factor: %
      mask Callback Offset: %
  EVT_Component : Outport  VectorParamsAs1DForOutWhenUnconnected=off
  EVT_Pack : Outport  Port=2  VectorParamsAs1DForOutWhenUnconnected=off
  EVT_ErrNr_CSC_16_Master : Outport  Port=3  VectorParamsAs1DForOutWhenUnconnected=off
  EVT_ErrNr_CSC_15_Master : Outport  Port=4  VectorParamsAs1DForOutWhenUnconnected=off
  EVT_ErrNr_CSC_14_Master : Outport  Port=5  VectorParamsAs1DForOutWhenUnconnected=off
  EVT_ErrNr_CSC_13_Master : Outport  Port=6  VectorParamsAs1DForOutWhenUnconnected=off
  EVT_ErrNr_CSC_12_Master : Outport  Port=7  VectorParamsAs1DForOutWhenUnconnected=off
  EVT_ErrNr_CSC_11_Master : Outport  Port=8  VectorParamsAs1DForOutWhenUnconnected=off
  EVT_ErrNr_CSC_09_Master : Outport  Port=9  VectorParamsAs1DForOutWhenUnconnected=off
  EVT_ErrNr_SC_Master : Outport  Port=10  VectorParamsAs1DForOutWhenUnconnected=off
  EVT_ErrNr_PMB_Master : Outport  Port=11  VectorParamsAs1DForOutWhenUnconnected=off
  EVT_ErrNr_CSC_10_Master : Outport  Port=12  VectorParamsAs1DForOutWhenUnconnected=off
  EVT_ErrNr_CSC_08_Master : Outport  Port=13  VectorParamsAs1DForOutWhenUnconnected=off
  EVT_ErrNr_CSC_07_Master : Outport  Port=14  VectorParamsAs1DForOutWhenUnconnected=off
  EVT_ErrNr_CSC_06_Master : Outport  Port=15  VectorParamsAs1DForOutWhenUnconnected=off
  EVT_ErrNr_CSC_05_Master : Outport  Port=16  VectorParamsAs1DForOutWhenUnconnected=off
  EVT_ErrNr_CSC_04_Master : Outport  Port=17  VectorParamsAs1DForOutWhenUnconnected=off
  EVT_ErrNr_CSC_03_Master : Outport  Port=18  VectorParamsAs1DForOutWhenUnconnected=off
  EVT_ErrNr_CSC_02_Master : Outport  Port=19  VectorParamsAs1DForOutWhenUnconnected=off
  EVT_ErrNr_MC_Master : Outport  Port=20  VectorParamsAs1DForOutWhenUnconnected=off
  EVT_ErrNr_CSC_01_Master : Outport  Port=21  VectorParamsAs1DForOutWhenUnconnected=off
  EVT_Context : Outport  Port=22  VectorParamsAs1DForOutWhenUnconnected=off
  EVT_Categorie_Master : Outport  Port=23  VectorParamsAs1DForOutWhenUnconnected=off
  EVT_Timer_Master : Outport  Port=24  VectorParamsAs1DForOutWhenUnconnected=off
  ErrorCode : Outport  Port=25  VectorParamsAs1DForOutWhenUnconnected=off
  wires:
  IO_CAN_ReadMsg/3 -> Terminator8/1
  IO_CAN_ReadMsg/4 -> Terminator7/1
  IO_CAN_ReadMsg/5 -> Terminator6/1
  IO_CAN_ConfigMsg/2(handle) -> IO_CAN_ReadMsg/1
  IO_CAN_ConfigMsg/1(ErrorCode) -> Terminator2/1
  IO_CAN_ReadMsg/1 -> ErrorCode/1
  IO_CAN_ReadMsg/2 -> bit_unpacking1/1(Data_in), bit_unpacking2/1(Data_in), bit_unpacking3/1(Data_in), bit_unpacking4/1(Data_in), bit_unpacking5/1(Data_in), bit_unpacking6/1(Data_in), bit_unpacking7/1(Data_in), bit_unpacking8/1(Data_in), bit_unpacking9/1(Data_in), bit_unpacking10/1(Data_in), bit_unpacking11/1(Data_in), bit_unpacking12/1(Data_in), bit_unpacking13/1(Data_in), bit_unpacking14/1(Data_in), bit_unpacking15/1(Data_in), bit_unpacking16/1(Data_in), bit_unpacking17/1(Data_in), bit_unpacking18/1(Data_in), bit_unpacking19/1(Data_in), bit_unpacking20/1(Data_in), bit_unpacking21/1(Data_in), bit_unpacking22/1(Data_in), bit_unpacking23/1(Data_in), bit_unpacking24/1(Data_in)
  bit_unpacking1/1(Data_out) -> EVT_Component/1
  bit_unpacking2/1(Data_out) -> EVT_Pack/1
  bit_unpacking3/1(Data_out) -> EVT_ErrNr_CSC_16_Master/1
  bit_unpacking4/1(Data_out) -> EVT_ErrNr_CSC_15_Master/1
  bit_unpacking5/1(Data_out) -> EVT_ErrNr_CSC_14_Master/1
  bit_unpacking6/1(Data_out) -> EVT_ErrNr_CSC_13_Master/1
  bit_unpacking7/1(Data_out) -> EVT_ErrNr_CSC_12_Master/1
  bit_unpacking8/1(Data_out) -> EVT_ErrNr_CSC_11_Master/1
  bit_unpacking9/1(Data_out) -> EVT_ErrNr_CSC_09_Master/1
  bit_unpacking10/1(Data_out) -> EVT_ErrNr_SC_Master/1
  bit_unpacking11/1(Data_out) -> EVT_ErrNr_PMB_Master/1
  bit_unpacking12/1(Data_out) -> EVT_ErrNr_CSC_10_Master/1
  bit_unpacking13/1(Data_out) -> EVT_ErrNr_CSC_08_Master/1
  bit_unpacking14/1(Data_out) -> EVT_ErrNr_CSC_07_Master/1
  bit_unpacking15/1(Data_out) -> EVT_ErrNr_CSC_06_Master/1
  bit_unpacking16/1(Data_out) -> EVT_ErrNr_CSC_05_Master/1
  bit_unpacking17/1(Data_out) -> EVT_ErrNr_CSC_04_Master/1
  bit_unpacking18/1(Data_out) -> EVT_ErrNr_CSC_03_Master/1
  bit_unpacking19/1(Data_out) -> EVT_ErrNr_CSC_02_Master/1
  bit_unpacking20/1(Data_out) -> EVT_ErrNr_MC_Master/1
  bit_unpacking21/1(Data_out) -> EVT_ErrNr_CSC_01_Master/1
  bit_unpacking22/1(Data_out) -> EVT_Context/1
  bit_unpacking23/1(Data_out) -> EVT_Categorie_Master/1
  bit_unpacking24/1(Data_out) -> EVT_Timer_Master/1
